simulink model "ClusterPositionControlInClusterSpace"  (R2016b)
settings: Solver=VariableStepAuto  StartTime=0.0  StopTime=100  RelTol=1e-3
libraries: simulink x1
settings Model: Creator=Zikinkeria  LastModifiedBy=Zikinkeria

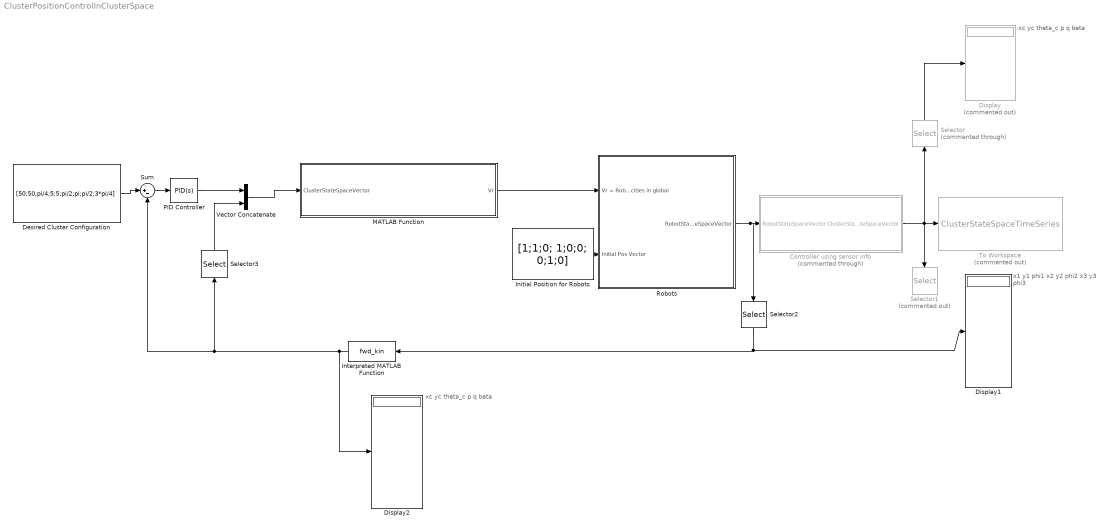
== system ClusterPositionControlInClusterSpace ==
  note: x1
      | y1
      | phi1
      | x2
      | y2
      | phi2
      | x3
      | y3
      | phi3
  note: xc
      | yc
      | theta_c
      | p
      | q
      | beta
  note: xc
      | yc
      | theta_c
      | p
      | q
      | beta
  Controller using sensor info : Subsystem  Commented=through
  Desired Cluster Configuration : Constant  Value=[50;50;pi/4;5;5;pi/2;pi;pi/2;3*pi/4]  VectorParams1D=off
  Display : Display  Commented=on
  Display1 : Display
  Display2 : Display
  Initial Position for Robots : Constant  Value=[1;1;0; 1;0;0; 0;1;0]  VectorParams1D=off
  Interpreted MATLAB Function : MATLABFcn  MATLABFcn=fwd_kin
  MATLAB Function : MATLAB Function  TreatAsAtomicUnit=on
  PID Controller : simulink/Continuous/PID Controller  Controller=PID  TimeDomain=Continuous-time  SampleTime=-1  IntegratorMethod=Forward Euler  FilterMethod=Forward Euler  Form=Parallel  UseFilter=on  ControllerParametersSource=internal  P=.1  I=0  D=0  N=100  InitialConditionSource=internal  InitialConditionForIntegrator=0  InitialConditionForFilter=0  ExternalReset=none  LimitOutput=off  UpperSaturationLimit=inf  LowerSaturationLimit=-inf  LinearizeAsGain=on  AntiWindupMode=none  Kb=1  TrackingMode=off  Kt=1  PParamMin=[]  PParamMax=[]  IParamMin=[]  IParamMax=[]  DParamMin=[]  DParamMax=[]  NParamMin=[]  NParamMax=[]  KbParamMin=[]  KbParamMax=[]  KtParamMin=[]  KtParamMax=[]  POutMin=[]  POutMax=[]  IOutMin=[]  IOutMax=[]  DOutMin=[]  DOutMax=[]  NOutMin=[]  NOutMax=[]  KbOutMin=[]  KbOutMax=[]  KtOutMin=[]  KtOutMax=[]  IntegratorOutMin=[]  IntegratorOutMax=[]  FilterOutMin=[]  FilterOutMax=[]  SumOutMin=[]  SumOutMax=[]  SumI1OutMin=[]  SumI1OutMax=[]  SumI2OutMin=[]  SumI2OutMax=[]  SumI3OutMin=[]  SumI3OutMax=[]  SumDOutMin=[]  SumDOutMax=[]  SaturationOutMin=[]  SaturationOutMax=[]  IntegratorContinuousStateAttributes=''  IntegratorStateMustResolveToSignalObject=off  IntegratorRTWStateStorageClass=Auto  FilterContinuousStateAttributes=''  FilterStateMustResolveToSignalObject=off  FilterRTWStateStorageClass=Auto  DifferentiatorICPrevScaledInput=0  DifferentiatorOutMin=[]  DifferentiatorOutMax=[]
  Robots : Subsystem
  Selector : Selector  Commented=through  InputPortWidth=26  IndexOptions=Index vector (dialog)  Indices=[16 17 18 19 20 21]  OutputSizes=1
  Selector1 : Selector  Commented=on  InputPortWidth=26  IndexOptions=Index vector (dialog)  Indices=[7, 8, 9, 10, 11, 12, 13, 14, 15]  OutputSizes=1
  Selector2 : Selector  InputPortWidth=18  IndexOptions=Index vector (dialog)  Indices=[1 2 3 4 5 6 7 8 9]  OutputSizes=1
  Selector3 : Selector  InputPortWidth=9  IndexOptions=Index vector (dialog)  Indices=[3 4 5 6]  OutputSizes=1
  Sum : Sum  Inputs=|+-
  To Workspace : ToWorkspace  Commented=on  VariableName=ClusterStateSpaceTimeSeries  SaveFormat=Timeseries  SampleTime=-1
  Vector Concatenate : Concatenate
  wires:
  Initial Position for Robots/1 -> Robots/2(Initial Pos Vector)
  Robots/1(RobotStateSpaceVector) -> Selector2/1, Controller using sensor info/1(RobotStateSpaceVector)
  Controller using sensor info/1(ClusterStateSpaceVector) -> Selector1/1, Selector/1, To Workspace/1
  Selector/1 -> Display/1
  Sum/1 -> PID Controller/1
  Desired Cluster Configuration/1 -> Sum/1
  Selector2/1 -> Interpreted MATLAB Function/1, Display1/1
  MATLAB Function/1(Vr) -> Robots/1(Vr = Robot Velocities in global)
  Interpreted MATLAB Function/1 -> Display2/1, Selector3/1, Sum/2
  PID Controller/1 -> Vector Concatenate/1
  Vector Concatenate/1 -> MATLAB Function/1(ClusterStateSpaceVector)
  Selector3/1 -> Vector Concatenate/2

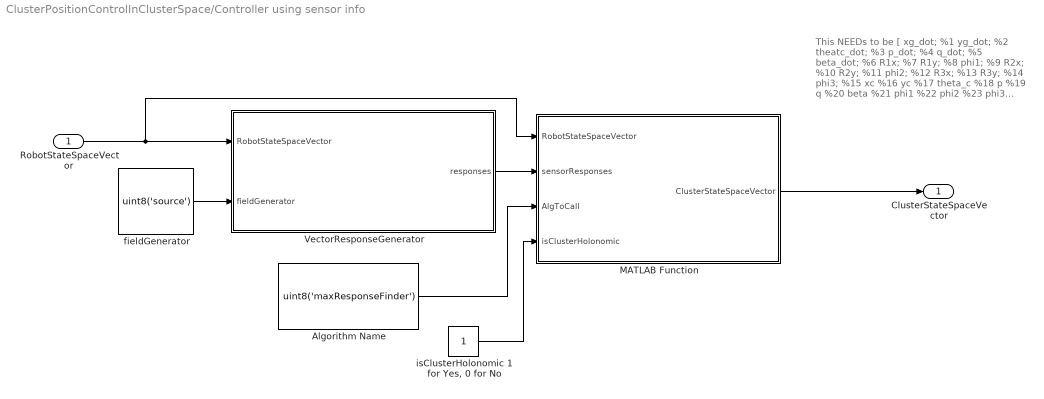
== system ClusterPositionControlInClusterSpace/Controller using sensor info ==
  note: This NEEDs to be
      | [
      |         xg_dot;         %1
      |         yg_dot;         %2
      |         theatc_dot;   %3
      |         p_dot;           %4
      |         q_dot;           %5
      |         beta_dot;      %6
      |         R1x;              %7
      |         R1y;              %8
      |         phi1;              %9
      |         R2x;              %10
      |         R2y;              %11
      |         phi2;              %12
      |         R3x;              %13
      |         R3y;              %14
      |         phi3;              %15
      |         xc                  %16
      |         yc                  %17
      |         theta_c          %18
      |         p                    %19
      |         q                    %20
      |         beta               %21
      |         phi1               %22
      |         phi2               %23
      |         phi3               %24
      |         xc_dot;          %25
      |         yc_dot;          %26
      |         ];
  RobotStateSpaceVector : Inport
  Algorithm Name : Constant  Value=uint8('maxResponseFinder')
  MATLAB Function : MATLAB Function  TreatAsAtomicUnit=on
  VectorResponseGenerator : MATLAB Function  TreatAsAtomicUnit=on
  fieldGenerator : Constant  Value=uint8('source')
  "isClusterHolonomic 1 for Yes, 0 for No" : Constant
  ClusterStateSpaceVector : Outport
  wires:
  fieldGenerator/1 -> VectorResponseGenerator/2(fieldGenerator)
  RobotStateSpaceVector/1 -> MATLAB Function/1(RobotStateSpaceVector), VectorResponseGenerator/1(RobotStateSpaceVector)
  Algorithm Name/1 -> MATLAB Function/3(AlgToCall)
  MATLAB Function/1(ClusterStateSpaceVector) -> ClusterStateSpaceVector/1
  VectorResponseGenerator/1(responses) -> MATLAB Function/2(sensorResponses)
  "isClusterHolonomic 1 for Yes, 0 for No"/1 -> MATLAB Function/4(isClusterHolonomic)

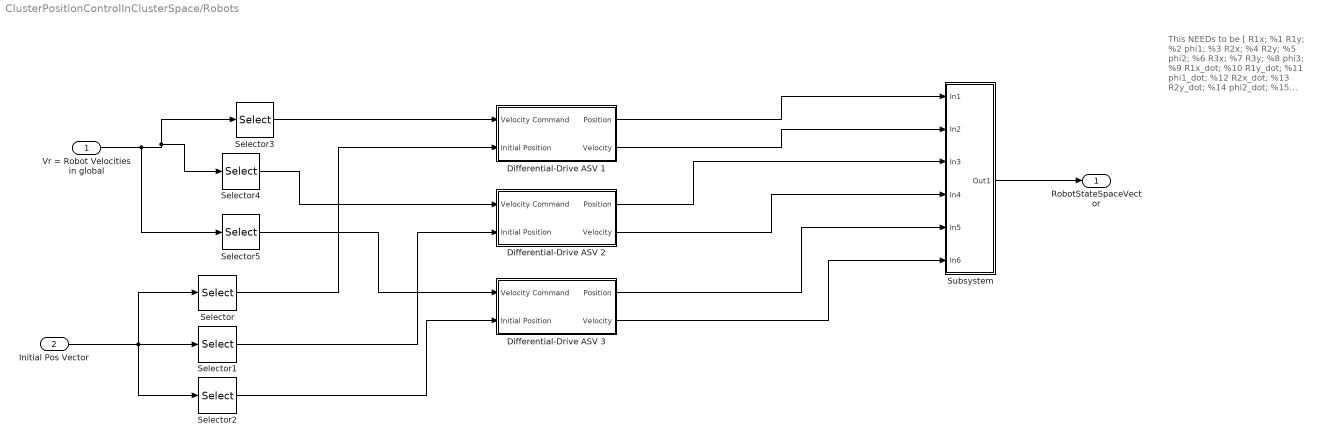
== system ClusterPositionControlInClusterSpace/Robots ==
  note: This NEEDs to be
      | [ R1x;        %1
      |   R1y;        %2
      |   phi1;        %3
      |   R2x;         %4
      |   R2y;         %5
      |   phi2;        %6
      |   R3x;         %7
      |   R3y;         %8
      |   phi3;         %9
      |   R1x_dot;  %10
      |   R1y_dot;  %11
      |   phi1_dot;  %12
      |   R2x_dot;  %13
      |   R2y_dot;  %14
      |   phi2_dot;  %15
      |   R3x_dot;  %16
      |   R3y_dot;  %17
      |   phi3_dot]; %18
      |
      | all in the global frame
  Vr = Robot Velocities in global : Inport
  Initial Pos Vector : Inport  Port=2
  Differential-Drive ASV 1 : Subsystem
  Differential-Drive ASV 2 : Subsystem
  Differential-Drive ASV 3 : Subsystem
  Selector : Selector  InputPortWidth=9  IndexOptions=Index vector (dialog)  Indices=[1 2 3]  OutputSizes=1
  Selector1 : Selector  InputPortWidth=9  IndexOptions=Index vector (dialog)  Indices=[4 5 6]  OutputSizes=1
  Selector2 : Selector  InputPortWidth=9  IndexOptions=Index vector (dialog)  Indices=[7 8 9]  OutputSizes=1
  Selector3 : Selector  InputPortWidth=9  IndexOptions=Index vector (dialog)  Indices=[1 2 3]  OutputSizes=1
  Selector4 : Selector  InputPortWidth=9  IndexOptions=Index vector (dialog)  Indices=[4 5 6]  OutputSizes=1
  Selector5 : Selector  InputPortWidth=9  IndexOptions=Index vector (dialog)  Indices=[7 8 9]  OutputSizes=1
  Subsystem : Subsystem
  RobotStateSpaceVector : Outport
  wires:
  Selector4/1 -> Differential-Drive ASV 2/1(Velocity Command)
  Selector5/1 -> Differential-Drive ASV 3/1(Velocity Command)
  Selector2/1 -> Differential-Drive ASV 3/2(Initial Position)
  Selector1/1 -> Differential-Drive ASV 2/2(Initial Position)
  Initial Pos Vector/1 -> Selector/1, Selector2/1, Selector1/1
  Selector/1 -> Differential-Drive ASV 1/2(Initial Position)
  Differential-Drive ASV 1/1(Position) -> Subsystem/1(In1)
  Differential-Drive ASV 1/2(Velocity) -> Subsystem/2(In2)
  Differential-Drive ASV 2/1(Position) -> Subsystem/3(In3)
  Differential-Drive ASV 2/2(Velocity) -> Subsystem/4(In4)
  Differential-Drive ASV 3/1(Position) -> Subsystem/5(In5)
  Differential-Drive ASV 3/2(Velocity) -> Subsystem/6(In6)
  Subsystem/1(Out1) -> RobotStateSpaceVector/1
  Selector3/1 -> Differential-Drive ASV 1/1(Velocity Command)
  Vr = Robot Velocities in global/1 -> Selector4/1, Selector3/1, Selector5/1

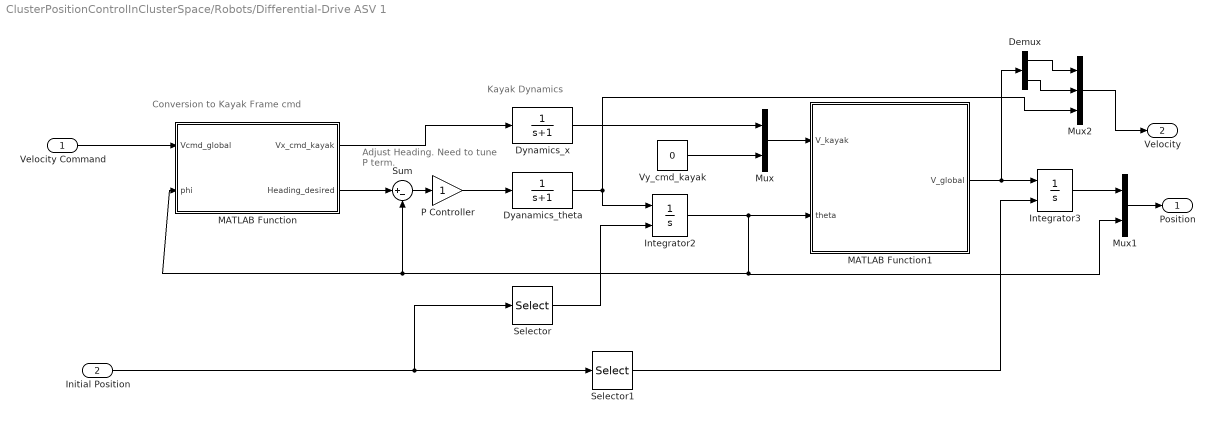
== system ClusterPositionControlInClusterSpace/Robots/Differential-Drive ASV 1 ==
  note: Conversion to Kayak Frame cmd
  note: Kayak Dynamics
  note: Adjust Heading. Need to tune P term.
  Velocity Command : Inport
  Initial Position : Inport  Port=2
  Demux : Demux  Outputs=2
  Dyanamics_theta : TransferFcn  Denominator=[1 1]
  Dynamics_x : TransferFcn  Denominator=[1 1]
  Integrator2 : Integrator  InitialConditionSource=external
  Integrator3 : Integrator  InitialConditionSource=external
  MATLAB Function : MATLAB Function  TreatAsAtomicUnit=on
  MATLAB Function1 : MATLAB Function  TreatAsAtomicUnit=on
  Mux : Mux  Inputs=2
  Mux1 : Mux  Inputs=2
  Mux2 : Mux  Inputs=3
  P Controller : Gain
  Selector : Selector  InputPortWidth=3  IndexOptions=Index vector (dialog)  Indices=[3]  OutputSizes=1
  Selector1 : Selector  InputPortWidth=3  IndexOptions=Index vector (dialog)  Indices=[1 2]  OutputSizes=1
  Sum : Sum  Inputs=|+-
  Vy_cmd_kayak : Constant  Value=0
  Position : Outport
  Velocity : Outport  Port=2
  wires:
  MATLAB Function/1(Vx_cmd_kayak) -> Dynamics_x/1
  MATLAB Function/2(Heading_desired) -> Sum/1
  Sum/1 -> P Controller/1
  P Controller/1 -> Dyanamics_theta/1
  Dyanamics_theta/1 -> Mux2/3, Integrator2/1
  Initial Position/1 -> Selector1/1, Selector/1
  Mux/1 -> MATLAB Function1/1(V_kayak)
  Dynamics_x/1 -> Mux/1
  Vy_cmd_kayak/1 -> Mux/2
  Integrator2/1 -> MATLAB Function/2(phi), Sum/2, Mux1/2, MATLAB Function1/2(theta)
  MATLAB Function1/1(V_global) -> Demux/1, Integrator3/1
  Selector/1 -> Integrator2/2
  Selector1/1 -> Integrator3/2
  Mux1/1 -> Position/1
  Integrator3/1 -> Mux1/1
  Demux/1 -> Mux2/1
  Demux/2 -> Mux2/2
  Mux2/1 -> Velocity/1
  Velocity Command/1 -> MATLAB Function/1(Vcmd_global)

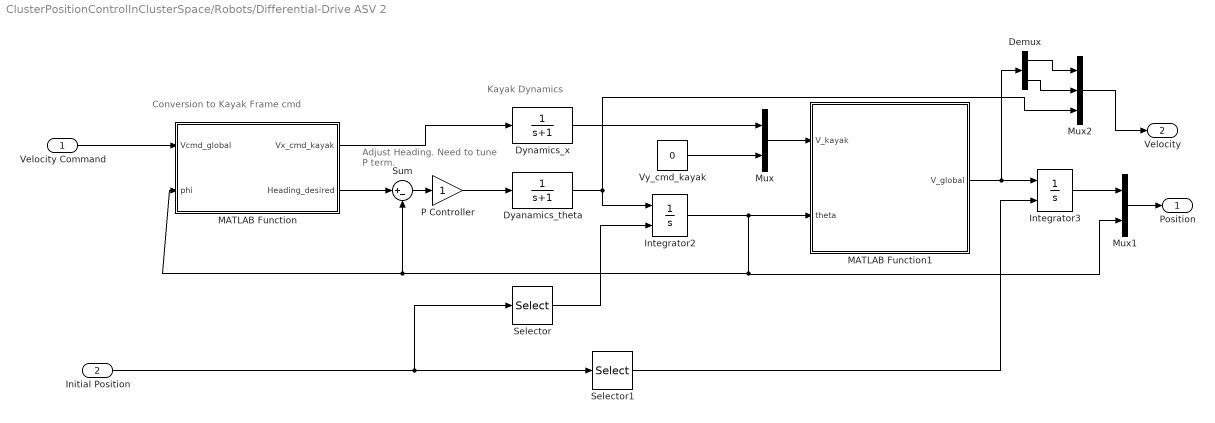
== system ClusterPositionControlInClusterSpace/Robots/Differential-Drive ASV 2 ==
  note: Conversion to Kayak Frame cmd
  note: Kayak Dynamics
  note: Adjust Heading. Need to tune P term.
  Velocity Command : Inport
  Initial Position : Inport  Port=2
  Demux : Demux  Outputs=2
  Dyanamics_theta : TransferFcn  Denominator=[1 1]
  Dynamics_x : TransferFcn  Denominator=[1 1]
  Integrator2 : Integrator  InitialConditionSource=external
  Integrator3 : Integrator  InitialConditionSource=external
  MATLAB Function : MATLAB Function  TreatAsAtomicUnit=on
  MATLAB Function1 : MATLAB Function  TreatAsAtomicUnit=on
  Mux : Mux  Inputs=2
  Mux1 : Mux  Inputs=2
  Mux2 : Mux  Inputs=3
  P Controller : Gain
  Selector : Selector  InputPortWidth=3  IndexOptions=Index vector (dialog)  Indices=[3]  OutputSizes=1
  Selector1 : Selector  InputPortWidth=3  IndexOptions=Index vector (dialog)  Indices=[1 2]  OutputSizes=1
  Sum : Sum  Inputs=|+-
  Vy_cmd_kayak : Constant  Value=0
  Position : Outport
  Velocity : Outport  Port=2
  wires:
  MATLAB Function/1(Vx_cmd_kayak) -> Dynamics_x/1
  MATLAB Function/2(Heading_desired) -> Sum/1
  Sum/1 -> P Controller/1
  P Controller/1 -> Dyanamics_theta/1
  Dyanamics_theta/1 -> Mux2/3, Integrator2/1
  Initial Position/1 -> Selector1/1, Selector/1
  Mux/1 -> MATLAB Function1/1(V_kayak)
  Dynamics_x/1 -> Mux/1
  Vy_cmd_kayak/1 -> Mux/2
  Integrator2/1 -> MATLAB Function/2(phi), Sum/2, Mux1/2, MATLAB Function1/2(theta)
  MATLAB Function1/1(V_global) -> Demux/1, Integrator3/1
  Selector/1 -> Integrator2/2
  Selector1/1 -> Integrator3/2
  Mux1/1 -> Position/1
  Integrator3/1 -> Mux1/1
  Demux/1 -> Mux2/1
  Demux/2 -> Mux2/2
  Mux2/1 -> Velocity/1
  Velocity Command/1 -> MATLAB Function/1(Vcmd_global)

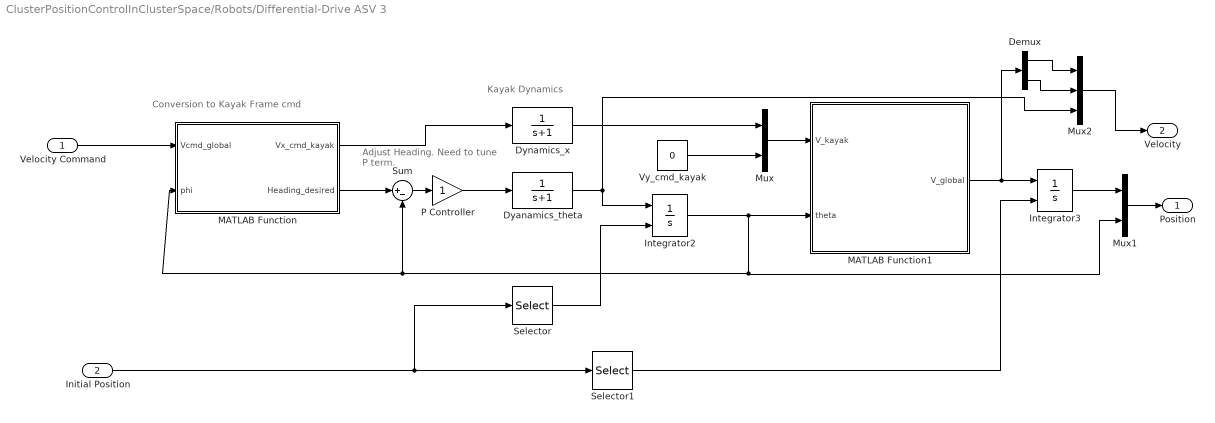
== system ClusterPositionControlInClusterSpace/Robots/Differential-Drive ASV 3 ==
  note: Conversion to Kayak Frame cmd
  note: Kayak Dynamics
  note: Adjust Heading. Need to tune P term.
  Velocity Command : Inport
  Initial Position : Inport  Port=2
  Demux : Demux  Outputs=2
  Dyanamics_theta : TransferFcn  Denominator=[1 1]
  Dynamics_x : TransferFcn  Denominator=[1 1]
  Integrator2 : Integrator  InitialConditionSource=external
  Integrator3 : Integrator  InitialConditionSource=external
  MATLAB Function : MATLAB Function  TreatAsAtomicUnit=on
  MATLAB Function1 : MATLAB Function  TreatAsAtomicUnit=on
  Mux : Mux  Inputs=2
  Mux1 : Mux  Inputs=2
  Mux2 : Mux  Inputs=3
  P Controller : Gain
  Selector : Selector  InputPortWidth=3  IndexOptions=Index vector (dialog)  Indices=[3]  OutputSizes=1
  Selector1 : Selector  InputPortWidth=3  IndexOptions=Index vector (dialog)  Indices=[1 2]  OutputSizes=1
  Sum : Sum  Inputs=|+-
  Vy_cmd_kayak : Constant  Value=0
  Position : Outport
  Velocity : Outport  Port=2
  wires:
  MATLAB Function/1(Vx_cmd_kayak) -> Dynamics_x/1
  MATLAB Function/2(Heading_desired) -> Sum/1
  Sum/1 -> P Controller/1
  P Controller/1 -> Dyanamics_theta/1
  Dyanamics_theta/1 -> Mux2/3, Integrator2/1
  Initial Position/1 -> Selector1/1, Selector/1
  Mux/1 -> MATLAB Function1/1(V_kayak)
  Dynamics_x/1 -> Mux/1
  Vy_cmd_kayak/1 -> Mux/2
  Integrator2/1 -> MATLAB Function/2(phi), Sum/2, Mux1/2, MATLAB Function1/2(theta)
  MATLAB Function1/1(V_global) -> Demux/1, Integrator3/1
  Selector/1 -> Integrator2/2
  Selector1/1 -> Integrator3/2
  Mux1/1 -> Position/1
  Integrator3/1 -> Mux1/1
  Demux/1 -> Mux2/1
  Demux/2 -> Mux2/2
  Mux2/1 -> Velocity/1
  Velocity Command/1 -> MATLAB Function/1(Vcmd_global)

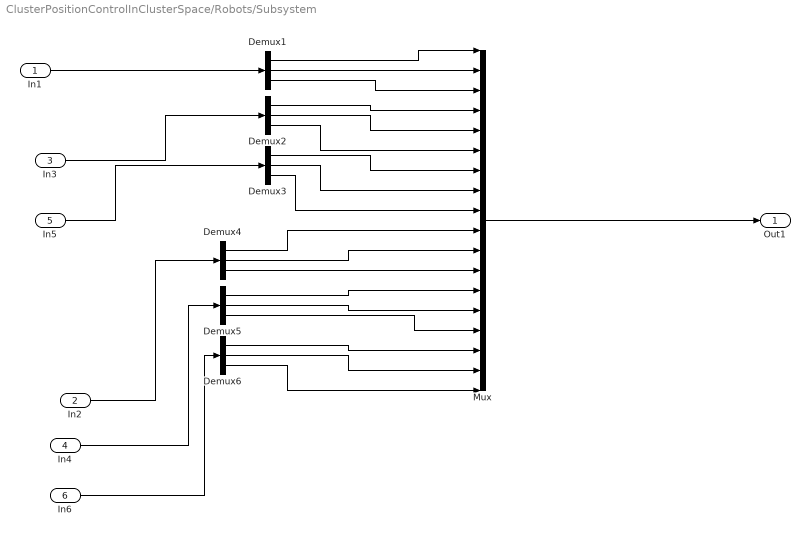
== system ClusterPositionControlInClusterSpace/Robots/Subsystem ==
  In1 : Inport
  In2 : Inport  Port=2
  In3 : Inport  Port=3
  In4 : Inport  Port=4
  In5 : Inport  Port=5
  In6 : Inport  Port=6
  Demux{1..6} (6 alike) : Demux  Outputs=3
  Mux : Mux  Inputs=18
  Out1 : Outport
  wires:
  Demux5/2 -> Mux/14
  Demux2/1 -> Mux/4
  Demux2/2 -> Mux/5
  Demux4/3 -> Mux/12
  Demux3/3 -> Mux/9
  Demux6/3 -> Mux/18
  Demux3/2 -> Mux/8
  Demux5/1 -> Mux/13
  Demux4/2 -> Mux/11
  Demux1/3 -> Mux/3
  Demux2/3 -> Mux/6
  Demux1/2 -> Mux/2
  Demux4/1 -> Mux/10
  Demux3/1 -> Mux/7
  Demux1/1 -> Mux/1
  Demux6/2 -> Mux/17
  Demux5/3 -> Mux/15
  Demux6/1 -> Mux/16
  In1/1 -> Demux1/1
  In4/1 -> Demux5/1
  In2/1 -> Demux4/1
  In3/1 -> Demux2/1
  In5/1 -> Demux3/1
  In6/1 -> Demux6/1
  Mux/1 -> Out1/1

== matlab function ClusterPositionControlInClusterSpace/Robots/Differential-Drive ASV 2/MATLAB Function ==
  data: Vcmd_global input; Vx_cmd_kayak output; Heading_desired output; phi input
function [Vx_cmd_kayak,Heading_desired] = fcn(Vcmd_global, phi)
Vx_cmd_global = Vcmd_global(1);
Vy_cmd_global = Vcmd_global(2);

Heading_desired = atan2(Vy_cmd_global,Vx_cmd_global);
Vx_cmd_kayak = sqrt(Vx_cmd_global^2 + Vy_cmd_global^2)*cos(abs(Heading_desired-phi));

== matlab function ClusterPositionControlInClusterSpace/Robots/Differential-Drive ASV 2/MATLAB Function1 ==
  data: V_kayak input; V_global output; theta input
function V_global = Robot_to_Frame_Transformation(V_kayak,theta)
%This function calculates the local robot velocities
%based on the global robot velocities

%Initialize Variables
V_robot = [V_kayak(1);V_kayak(2)];

T = [cos(theta) -sin(theta);...
    sin(theta) cos(theta)];
V_global = T*V_robot;

== matlab function ClusterPositionControlInClusterSpace/Robots/Differential-Drive ASV 3/MATLAB Function ==
  data: Vcmd_global input; Vx_cmd_kayak output; Heading_desired output; phi input
function [Vx_cmd_kayak,Heading_desired] = fcn(Vcmd_global, phi)
Vx_cmd_global = Vcmd_global(1);
Vy_cmd_global = Vcmd_global(2);

Heading_desired = atan2(Vy_cmd_global,Vx_cmd_global);
Vx_cmd_kayak = sqrt(Vx_cmd_global^2 + Vy_cmd_global^2)*cos(abs(Heading_desired-phi));

== matlab function ClusterPositionControlInClusterSpace/MATLAB Function ==
  data: ClusterStateSpaceVector input; Vr output

function Vr = inverse_jacobian( ClusterStateSpaceVector )
%INVERSE_JACOBIAN Returns the inverse jacobian
%   This is for a three bot p,q,beta cluster, in aero frame
%disp(ClusterStateSpaceVector);
% theta_c = ClusterStateSpaceVector(18);
% p = ClusterStateSpaceVector(19);
% q = ClusterStateSpaceVector(20);
% beta1 = ClusterStateSpaceVector(21);

theta_c = ClusterStateSpaceVector(10);
p = ClusterStateSpaceVector(11);
q = ClusterStateSpaceVector(12);
beta1 = ClusterStateSpaceVector(13);

disp('theta_c');
disp(theta_c);
disp('p');
disp(p);
disp('q');
disp(q);
disp('beta1');
disp(beta1);

inv_Jac = [ 1, 0, -(sin(theta_c)*(p^2 + 2*cos(beta1)*p*q + q^2)^(1/2))/3, (cos(theta_c)*(2*p + 2*q*cos(beta1)))/(6*(p^2 + 2*cos(beta1)*p*q + q^2)^(1/2)), (cos(theta_c)*(2*q + 2*p*cos(beta1)))/(6*(p^2 + 2*cos(beta1)*p*q + q^2)^(1/2)), -(p*q*sin(beta1)*cos(theta_c))/(3*(p^2 + 2*cos(beta1)*p*q + q^2)^(1/2)), 0, 0, 0;
 0, 1,  (cos(theta_c)*(p^2 + 2*cos(beta1)*p*q + q^2)^(1/2))/3, (sin(theta_c)*(2*p + 2*q*cos(beta1)))/(6*(p^2 + 2*cos(beta1)*p*q + q^2)^(1/2)), (sin(theta_c)*(2*q + 2*p*cos(beta1)))/(6*(p^2 + 2*cos(beta1)*p*q + q^2)^(1/2)), -(p*q*sin(beta1)*sin(theta_c))/(3*(p^2 + 2*cos(beta1)*p*q + q^2)^(1/2)), 0, 0, 0;
 0, 0, 1, 0, 0, 0, 1, 0, 0;
 1, 0, p*cos(theta_c)*(-(q^2*(cos(beta1)^2 - 1))/(p^2 + 2*cos(beta1)*p*q + q^2))^(1/2) + (sin(theta_c)*(2*p^2 + cos(beta1)*p*q - q^2))/(3*(p^2 + 2*cos(beta1)*p*q + q^2)^(1/2)),   sin(theta_c)*(-(q^2*(cos(beta1)^2 - 1))/(p^2 + 2*cos(beta1)*p*q + q^2))^(1/2) - (cos(theta_c)*(5*p*q^2 + 2*p^3 + 2*q^3*cos(beta1) + 6*p^2*q*cos(beta1) + p*q^2*cos(beta1)^2))/(3*(p^2 + 2*cos(beta1)*p*q + q^2)^(3/2)) + (p*q^2*sin(theta_c)*(p + q*cos(beta1))*(cos(beta1)^2 - 1))/((p^2 + 2*cos(beta1)*p*q + q^2)^2*(-(q^2*(cos(beta1)^2 - 1))/(p^2 + 2*cos(beta1)*p*q + q^2))^(1/2)), (cos(theta_c)*(4*p^2*q + q^3 + p^3*cos(beta1) + 3*p*q^2*cos(beta1) - p^2*q*cos(beta1)^2))/(3*(p^2 + 2*cos(beta1)*p*q + q^2)^(3/2)) - (p^2*q*sin(theta_c)*(p + q*cos(beta1))*(cos(beta1)^2 - 1))/((p^2 + 2*cos(beta1)*p*q + q^2)^2*(-(q^2*(cos(beta1)^2 - 1))/(p^2 + 2*cos(beta1)*p*q + q^2))^(1/2)), (p*q*sin(beta1)*cos(theta_c)*(- p^2 + cos(beta1)*p*q + 2*q^2))/(3*(p^2 + 2*cos(beta1)*p*q + q^2)^(3/2)) + (p*q^2*sin(beta1)*sin(theta_c)*(p^2*cos(beta1) + p*q*cos(beta1)^2 + p*q + q^2*cos(beta1)))/((p^2 + 2*cos(beta1)*p*q + q^2)^2*(-(q^2*(cos(beta1)^2 - 1))/(p^2 + 2*cos(beta1)*p*q + q^2))^(1/2)), 0, 0, 0;
 0, 1, p*sin(theta_c)*(-(q^2*(cos(beta1)^2 - 1))/(p^2 + 2*cos(beta1)*p*q + q^2))^(1/2) - (cos(theta_c)*(2*p^2 + cos(beta1)*p*q - q^2))/(3*(p^2 + 2*cos(beta1)*p*q + q^2)^(1/2)), - cos(theta_c)*(-(q^2*(cos(beta1)^2 - 1))/(p^2 + 2*cos(beta1)*p*q + q^2))^(1/2) - (sin(theta_c)*(5*p*q^2 + 2*p^3 + 2*q^3*cos(beta1) + 6*p^2*q*cos(beta1) + p*q^2*cos(beta1)^2))/(3*(p^2 + 2*cos(beta1)*p*q + q^2)^(3/2)) - (p*q^2*cos(theta_c)*(p + q*cos(beta1))*(cos(beta1)^2 - 1))/((p^2 + 2*cos(beta1)*p*q + q^2)^2*(-(q^2*(cos(beta1)^2 - 1))/(p^2 + 2*cos(beta1)*p*q + q^2))^(1/2)), (sin(theta_c)*(4*p^2*q + q^3 + p^3*cos(beta1) + 3*p*q^2*cos(beta1) - p^2*q*cos(beta1)^2))/(3*(p^2 + 2*cos(beta1)*p*q + q^2)^(3/2)) + (p^2*q*cos(theta_c)*(p + q*cos(beta1))*(cos(beta1)^2 - 1))/((p^2 + 2*cos(beta1)*p*q + q^2)^2*(-(q^2*(cos(beta1)^2 - 1))/(p^2 + 2*cos(beta1)*p*q + q^2))^(1/2)), (p*q*sin(beta1)*sin(theta_c)*(- p^2 + cos(beta1)*p*q + 2*q^2))/(3*(p^2 + 2*cos(beta1)*p*q + q^2)^(3/2)) - (p*q^2*sin(beta1)*cos(theta_c)*(p^2*cos(beta1) + p*q*cos(beta1)^2 + p*q + q^2*cos(beta1)))/((p^2 + 2*cos(beta1)*p*q + q^2)^2*(-(q^2*(cos(beta1)^2 - 1))/(p^2 + 2*cos(beta1)*p*q + q^2))^(1/2)), 0, 0, 0;
 0, 0, 1, 0, 0, 0, 0, 1, 0;
 1, 0, (sin(theta_c)*(- p^2 + cos(beta1)*p*q + 2*q^2))/(3*(p^2 + 2*cos(beta1)*p*q + q^2)^(1/2)) - q*cos(theta_c)*(-(p^2*(cos(beta1)^2 - 1))/(p^2 + 2*cos(beta1)*p*q + q^2))^(1/2),                                                                                       (cos(theta_c)*(4*p*q^2 + p^3 + q^3*cos(beta1) + 3*p^2*q*cos(beta1) - p*q^2*cos(beta1)^2))/(3*(p^2 + 2*cos(beta1)*p*q + q^2)^(3/2)) + (p*q^2*sin(theta_c)*(q + p*cos(beta1))*(cos(beta1)^2 - 1))/((p^2 + 2*cos(beta1)*p*q + q^2)^2*(-(p^2*(cos(beta1)^2 - 1))/(p^2 + 2*cos(beta1)*p*q + q^2))^(1/2)), - sin(theta_c)*(-(p^2*(cos(beta1)^2 - 1))/(p^2 + 2*cos(beta1)*p*q + q^2))^(1/2) - (cos(theta_c)*(5*p^2*q + 2*q^3 + 2*p^3*cos(beta1) + 6*p*q^2*cos(beta1) + p^2*q*cos(beta1)^2))/(3*(p^2 + 2*cos(beta1)*p*q + q^2)^(3/2)) - (p^2*q*sin(theta_c)*(q + p*cos(beta1))*(cos(beta1)^2 - 1))/((p^2 + 2*cos(beta1)*p*q + q^2)^2*(-(p^2*(cos(beta1)^2 - 1))/(p^2 + 2*cos(beta1)*p*q + q^2))^(1/2)),   (p*q*sin(beta1)*cos(theta_c)*(2*p^2 + cos(beta1)*p*q - q^2))/(3*(p^2 + 2*cos(beta1)*p*q + q^2)^(3/2)) - (p^2*q*sin(beta1)*sin(theta_c)*(p^2*cos(beta1) + p*q*cos(beta1)^2 + p*q + q^2*cos(beta1)))/((p^2 + 2*cos(beta1)*p*q + q^2)^2*(-(p^2*(cos(beta1)^2 - 1))/(p^2 + 2*cos(beta1)*p*q + q^2))^(1/2)), 0, 0, 0;
 0, 1, - q*sin(theta_c)*(-(p^2*(cos(beta1)^2 - 1))/(p^2 + 2*cos(beta1)*p*q + q^2))^(1/2) - (cos(theta_c)*(- p^2 + cos(beta1)*p*q + 2*q^2))/(3*(p^2 + 2*cos(beta1)*p*q + q^2)^(1/2)), (sin(theta_c)*(4*p*q^2 + p^3 + q^3*cos(beta1) + 3*p^2*q*cos(beta1) - p*q^2*cos(beta1)^2))/(3*(p^2 + 2*cos(beta1)*p*q + q^2)^(3/2)) - (p*q^2*cos(theta_c)*(q + p*cos(beta1))*(cos(beta1)^2 - 1))/((p^2 + 2*cos(beta1)*p*q + q^2)^2*(-(p^2*(cos(beta1)^2 - 1))/(p^2 + 2*cos(beta1)*p*q + q^2))^(1/2)),   cos(theta_c)*(-(p^2*(cos(beta1)^2 - 1))/(p^2 + 2*cos(beta1)*p*q + q^2))^(1/2) - (sin(theta_c)*(5*p^2*q + 2*q^3 + 2*p^3*cos(beta1) + 6*p*q^2*cos(beta1) + p^2*q*cos(beta1)^2))/(3*(p^2 + 2*cos(beta1)*p*q + q^2)^(3/2)) + (p^2*q*cos(theta_c)*(q + p*cos(beta1))*(cos(beta1)^2 - 1))/((p^2 + 2*cos(beta1)*p*q + q^2)^2*(-(p^2*(cos(beta1)^2 - 1))/(p^2 + 2*cos(beta1)*p*q + q^2))^(1/2)),   (p*q*sin(beta1)*sin(theta_c)*(2*p^2 + cos(beta1)*p*q - q^2))/(3*(p^2 + 2*cos(beta1)*p*q + q^2)^(3/2)) + (p^2*q*sin(beta1)*cos(theta_c)*(p^2*cos(beta1) + p*q*cos(beta1)^2 + p*q + q^2*cos(beta1)))/((p^2 + 2*cos(beta1)*p*q + q^2)^2*(-(p^2*(cos(beta1)^2 - 1))/(p^2 + 2*cos(beta1)*p*q + q^2))^(1/2)), 0, 0, 0;
 0, 0, 1, 0, 0, 0, 0, 0, 1];
%Vc = [xc_dot; yc_dot; theta_c_dot; p_dot; q_dot; beta_dot; phi1_dot; phi2_dot; phi3_dot];
% Vc = [ ClusterStateSpaceVector(25); % xc_dot        %1
%        ClusterStateSpaceVector(26); % yc_dot        %2
%        ClusterStateSpaceVector(3);  % thetac_dot    %3
%        ClusterStateSpaceVector(4);  % p_dot         %4
%        ClusterStateSpaceVector(5);  % beta_dot      %5
%        ClusterStateSpaceVector(6);  % q_dot         %6
%        ClusterStateSpaceVector(22); % phi1_dot      %7
%        ClusterStateSpaceVector(23); % phi2_dot      %8
%        ClusterStateSpaceVector(24)];% phi3_dot      %9
Vc = [ClusterStateSpaceVector(1);
    ClusterStateSpaceVector(2);
    ClusterStateSpaceVector(3);
    ClusterStateSpaceVector(4);
    ClusterStateSpaceVector(5);
    ClusterStateSpaceVector(6);
    ClusterStateSpaceVector(7);
    ClusterStateSpaceVector(8);
    ClusterStateSpaceVector(9);];
Vr = inv_Jac*Vc;
end

== matlab function ClusterPositionControlInClusterSpace/Robots/Differential-Drive ASV 1/MATLAB Function ==
  data: Vcmd_global input; Vx_cmd_kayak output; Heading_desired output; phi input
function [Vx_cmd_kayak,Heading_desired] = fcn(Vcmd_global, phi)
Vx_cmd_global = Vcmd_global(1);
Vy_cmd_global = Vcmd_global(2);

Heading_desired = atan2(Vy_cmd_global,Vx_cmd_global);
Vx_cmd_kayak = sqrt(Vx_cmd_global^2 + Vy_cmd_global^2)*cos(abs(Heading_desired-phi));

== matlab function ClusterPositionControlInClusterSpace/Robots/Differential-Drive ASV 1/MATLAB Function1 ==
  data: V_kayak input; V_global output; theta input
function V_global = Robot_to_Frame_Transformation(V_kayak,theta)
%This function calculates the local robot velocities
%based on the global robot velocities

%Initialize Variables
V_robot = [V_kayak(1);V_kayak(2)];

T = [cos(theta) -sin(theta);...
    sin(theta) cos(theta)];
V_global = T*V_robot;

== matlab function ClusterPositionControlInClusterSpace/Robots/Differential-Drive ASV 3/MATLAB Function1 ==
  data: V_kayak input; V_global output; theta input
function V_global = Robot_to_Frame_Transformation(V_kayak,theta)
%This function calculates the local robot velocities
%based on the global robot velocities

%Initialize Variables
V_robot = [V_kayak(1);V_kayak(2)];

T = [cos(theta) -sin(theta);...
    sin(theta) cos(theta)];
V_global = T*V_robot;

== matlab function ClusterPositionControlInClusterSpace/Controller using sensor info/MATLAB Function ==
  data: RobotStateSpaceVector input; ClusterStateSpaceVector output; sensorResponses input; AlgToCall input; isClusterHolonomic input
function ClusterStateSpaceVector = AlgorithmCaller(RobotStateSpaceVector, sensorResponses, AlgToCall, isClusterHolonomic)
    AlgToCall = char(AlgToCall);
    ClusterStateSpaceVector = zeros(26, 1);
    % Calls the function store in AlgToCall and handles creating the
    %RobotStateSpaceVector = [ 
    %    R1x;       %1
    %    R1y;       %2
    %    phi1;      %3
    %    R2x;       %4
    %    R2y;       %5
    %    phi2;      %6
    %    R3x;       %7
    %    R3y;       %8
    %    phi3;      %9
    %    R1x_dot;   %10
    %    R1y_dot;   %11
    %    phi1_dot;  %12
    %    R2x_dot;   %13
    %    R2y_dot;   %14
    %    phi2_dot;  %15
    %    R3x_dot;   %16
    %    R3y_dot;   %17
    %    phi3_dot]; %18
    r1_pos = RobotStateSpaceVector(1:3);
    r2_pos = RobotStateSpaceVector(4:6);
    r3_pos = RobotStateSpaceVector(7:9);
    
    g1_unit = feval(AlgToCall, r1_pos, r2_pos, r3_pos, sensorResponses);
    
    rVars = [r1_pos, r2_pos, r3_pos]; % verify this
    clusterVars = fwd_kin(rVars);
    clusterTheta = clusterVars(3);

    %Rotation matrix from global frame to cluster frame.
%      Rcg = [cos(clusterTheta), sin(clusterTheta), 0; 
%             -sin(clusterTheta), cos(clusterTheta), 0;
%             0, 0, 1];
    des_theta = 0;
    des_theta = atan2(g1_unit(2), g1_unit(1));
    thetac_dot = 0;
    thetac_dot = double(des_theta)-double(clusterTheta);
    p_dot = 0; %Can be used to change the size of the cluster
    q_dot = 0;
    beta_dot = 0;
    if isClusterHolonomic
       yc_dot = sin(des_theta);
       xc_dot = cos(des_theta);
    else
       yc_dot = 0;
       xc_dot = 1; % makes the command non holonomic
    end

    Rgc = [cos(clusterTheta), -sin(clusterTheta);
            sin(clusterTheta), cos(clusterTheta)];
       
    %Transformation into global frame
    vg_dot = Rgc*([xc_dot yc_dot]');
    xg_dot = vg_dot(1);
    yg_dot = vg_dot(2);
    
    ClusterStateSpaceVector = zeros(26,1);
    ClusterStateSpaceVector = [
        xg_dot;                                 %1
        yg_dot;                                 %2
        thetac_dot;                             %3
        p_dot;                                  %4
        q_dot;                                  %5
        beta_dot;                               %6
        r1_pos(1);                  %R1x        %7
        r1_pos(2);                  %R1y        %8
        r1_pos(3);                  %phi1       %9
        r2_pos(1);                  %R2x        %10
        r2_pos(2);                  %R2y        %11
        r2_pos(3);                  %phi2       %12
        r3_pos(1);                  %R3x        %13
        r3_pos(2);                  %R3y        %14
        r3_pos(3);                  %phi3       %15
        clusterVars(1);             %xc         %16
        clusterVars(2);             %yc         %17
        clusterVars(3);             %theta_c    %18
        clusterVars(4);             %p          %19
        clusterVars(5);             %q          %20
        clusterVars(6);             %beta       %21
        RobotStateSpaceVector(12);  %phi1_dot   %22
        RobotStateSpaceVector(15);  %phi2_dot   %23
        RobotStateSpaceVector(18);  %phi3_dot   %24
        xc_dot;                                 %25
        yc_dot;                                 %26
        ];
    %ClusterStateSpaceVector = ClusterStateSpaceVector';
end

== matlab function ClusterPositionControlInClusterSpace/Controller using sensor info/VectorResponseGenerator ==
  data: RobotStateSpaceVector input; responses output size=[3,2]; fieldGenerator input
function responses = VectorResponseGenerator(RobotStateSpaceVector, fieldGenerator)
    %RobotStateSpaceVector = [ 
    %    R1x;       %1
    %    R1y;       %2
    %    phi1;      %3
    %    R2x;       %4
    %    R2y;       %5
    %    phi2;      %6
    %    R3x;       %7
    %    R3y;       %8
    %    phi3;      %9
    %    R1x_dot;   %10
    %    R1y_dot;   %11
    %    phi1_dot;  %12
    %    R2x_dot;   %13
    %    R2y_dot;   %14
    %    phi2_dot;  %15
    %    R3x_dot;   %16
    %    R3y_dot;   %17
    %    phi3_dot]; %18
    fieldGenerator = char(fieldGenerator);
    R1 = feval(fieldGenerator, RobotStateSpaceVector(1), RobotStateSpaceVector(2));
    R2 = feval(fieldGenerator, RobotStateSpaceVector(4), RobotStateSpaceVector(5));
    R3 = feval(fieldGenerator, RobotStateSpaceVector(7), RobotStateSpaceVector(8));
    responses = zeros(3,2);
    responses = [R1; R2; R3];
end
